simulink library "AEB_L2"  (R2024b)
settings: Solver=VariableStepAuto  StartTime=0.0  StopTime=10.0  RelTol=1e-3

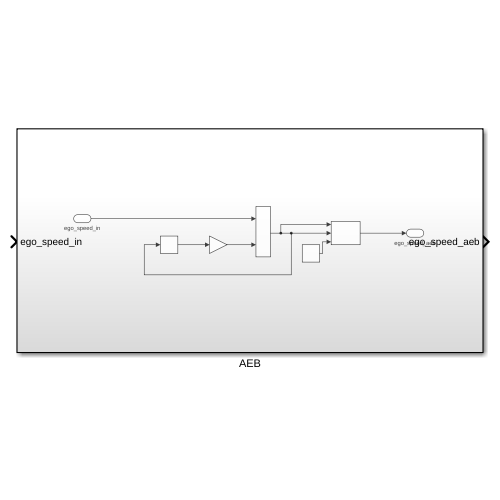
[thumbnail: Simulink's stored preview of the top-level diagram]
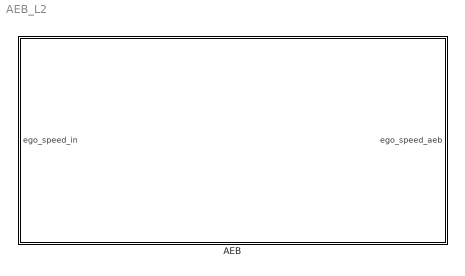
== system AEB_L2 ==
  AEB : Subsystem

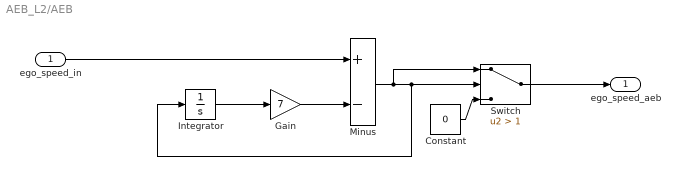
== system AEB_L2/AEB ==
  ego_speed_in : Inport
  Constant : Constant  Value=0
  Gain : Gain  Gain=7
  Integrator : Integrator
  Minus : Sum  Inputs=+-
  Switch : Switch  Criteria=u2 > Threshold  Threshold=1  SaturateOnIntegerOverflow=off  InputSameDT=off
  ego_speed_aeb : Outport
  wires:
  Gain/1 -> Minus/2
  Integrator/1 -> Gain/1
  Switch/1 -> ego_speed_aeb/1
  Minus/1 -> Switch/1, Integrator/1, Switch/2
  ego_speed_in/1 -> Minus/1
  Constant/1 -> Switch/3
